simulink model "select_function"  (R2019a)
settings: Solver=VariableStepAuto  StartTime=0.0  StopTime=10.0  RelTol=1e-3
settings Model: Creator=a3bawa  LastModifiedBy=a3bawa

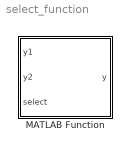
== system select_function ==
  MATLAB Function : MATLAB Function  TreatAsAtomicUnit=on

== matlab function select_function/MATLAB Function ==
  data: y1 input; y output; y2 input; select input
function y = fcn(y1,y2,select)

if select>=1
    y=y2;
else
    y=y1;
end
